simulink model "sampleModel209"  (R2021b)
settings: Solver=VariableStepAuto  StartTime=0.0  StopTime=10.0  RelTol=1e-3
undefined symbols (not defined in the file or in its folder): DiscIntNeverNeededParam, Newton, Raphson
libraries: simulink x2
settings Model: Creator=user  LastModifiedBy=user

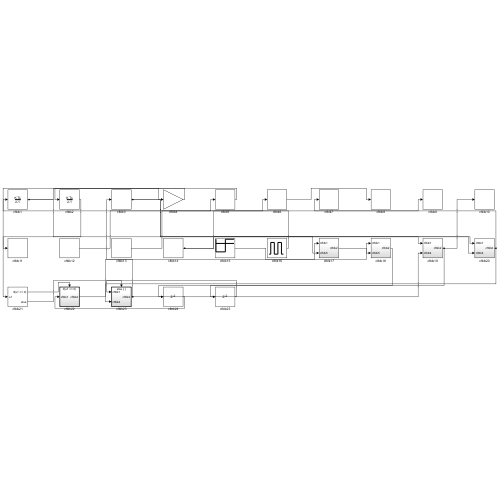
[thumbnail: Simulink's stored preview of the top-level diagram]
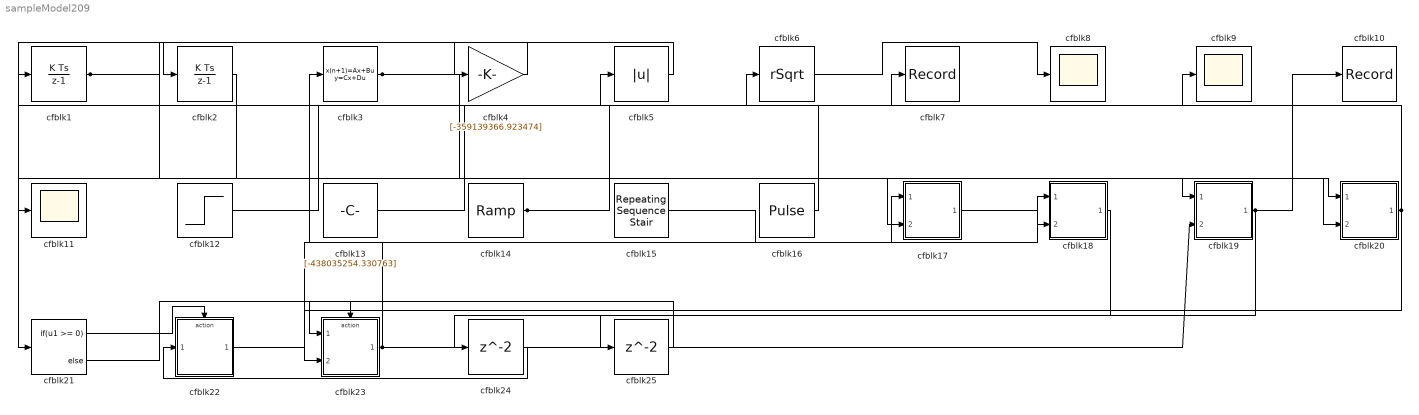
== system sampleModel209 ==
  cfblk1 : DiscreteIntegrator  ICPrevOutput=DiscIntNeverNeededParam  ICPrevScaledInput=DiscIntNeverNeededParam
  cfblk10 : Record  FileSettingsInternal="{\"entries\":[{\"content\":{\"excelSettings\":{\"content\":{},\"type\":\"Streamout.ExcelSettings\"}},\"type\":\"Streamout.FileSettingStorage\",\"uuid\":\"ddcee48c-97f9-4c5e-be8b-3015be74b49a\"}],\"packageUris\":[\"http://schema.mathworks.com/mf0/streamout_blocks/R2020a\"],\"version\":\"1.0\"}"  SignalsInternal="{\"entries\":[{\"content\":{\"signals\":[{\"content\":{\"blockPath\":[\"sampleModel209/cfblk10\"],\"channel\":[],\"dimensions\":[1],\"domain\":\"sampleModel209/cfblk10\",\"lineColor\":\"#ff13a6\",\"plots\":[1],\"port\":1,\"sid\":[\"\"],\"signalID\":8107,\"signalName\":\"cfblk19\"},\"type\":\"RecordBlkView.Signal\",\"uuid\":\"8c198879-0a60-44c0-909a-365ac949948a\"}]},\"type\":\"RecordBlkView.InputSignals\",\"uuid\":\"fa839402-d960-43c3-8ba2-43e0def371db\"}],\"packageUris\":[\"http://schema.mathworks.com/mf0/streamout_blocks/R2020a\"],\"version\":\"1.0\"}"  VisualizationBindings="{\"sparklinesplugin\":{\"info\":[{\"bindingParametersList\":[],\"subplotID\":1}]}}"
  cfblk11 : Scope
  cfblk12 : Step  Time=[34.000000]  Before=[760172402.159032]  After=[340434112.480645]  SampleTime=0
  cfblk13 : Constant  Value=[-438035254.330763]  SampleTime=1
  cfblk14 : simulink/Sources/Ramp  slope=[-6896.997594]  start=[40.335402]  InitialOutput=[-525774.390011]
  cfblk15 : simulink/Sources/Repeating Sequence Stair  OutValues=[-725082246.966305, 369090109.058846]  tsamp=-1  OutMin=[]  OutMax=[]  OutDataTypeStr=double  OutputDataTypeScalingMode=double  OutDataType=fixdt(0,8)  ConRadixGroup=Best Precision: Vector-wise  OutScaling=2^-12
  cfblk16 : DiscretePulseGenerator  PulseType=Time based  Amplitude=[-634459227.469684]  Period=[3400026.159223]  PulseWidth=5  PhaseDelay=[1.000000]
  cfblk17 : Subsystem
  cfblk18 : Subsystem
  cfblk19 : Subsystem
  cfblk2 : DiscreteIntegrator  ICPrevOutput=DiscIntNeverNeededParam  ICPrevScaledInput=DiscIntNeverNeededParam
  cfblk20 : Subsystem
  cfblk21 : If  IfExpression=u1 >= 0  SampleTime=1
  cfblk22 : Subsystem  TreatAsAtomicUnit=on
  cfblk23 : Subsystem  TreatAsAtomicUnit=on
  cfblk24 : Delay  SampleTime=1
  cfblk25 : Delay  SampleTime=1
  cfblk3 : DiscreteStateSpace
  cfblk4 : Gain  Gain=[-359139366.923474]
  cfblk5 : Abs
  cfblk6 : Sqrt  Operator=rSqrt  AlgorithmType=Newton-Raphson  SaturateOnIntegerOverflow=on
  cfblk7 : Record  FileSettingsInternal="{\"entries\":[{\"content\":{\"excelSettings\":{\"content\":{},\"type\":\"Streamout.ExcelSettings\"}},\"type\":\"Streamout.FileSettingStorage\",\"uuid\":\"78a27359-255d-4437-ae35-127f47ed64b3\"}],\"packageUris\":[\"http://schema.mathworks.com/mf0/streamout_blocks/R2020a\"],\"version\":\"1.0\"}"  SignalsInternal="{\"entries\":[{\"content\":{\"signals\":[{\"content\":{\"blockPath\":[\"sampleModel209/cfblk7\"],\"channel\":[],\"dimensions\":[1],\"domain\":\"sampleModel209/cfblk7\",\"lineColor\":\"#fe330a\",\"plots\":[1],\"port\":1,\"sid\":[\"\"],\"signalID\":8111,\"signalName\":\"cfblk20\"},\"type\":\"RecordBlkView.Signal\",\"uuid\":\"cc093a5e-f450-4358-995f-cba163aa30d8\"}]},\"type\":\"RecordBlkView.InputSignals\",\"uuid\":\"e5813685-5132-4ee3-bc5a-e7e5b18a0bcd\"}],\"packageUris\":[\"http://schema.mathworks.com/mf0/streamout_blocks/R2020a\"],\"version\":\"1.0\"}"  VisualizationBindings="{\"sparklinesplugin\":{\"info\":[{\"bindingParametersList\":[],\"subplotID\":1}]}}"
  cfblk8 : Scope
  cfblk9 : Scope
  wires:
  cfblk3/1 -> cfblk19/1(cfblk1), cfblk17/2(cfblk5)
  cfblk13/1 -> cfblk5/1
  cfblk5/1 -> cfblk21/1
  cfblk4/1 -> cfblk2/1
  cfblk15/1 -> cfblk18/1(cfblk1)
  cfblk17/1(cfblk2) -> cfblk18/2(cfblk5)
  cfblk20/1(cfblk2) -> cfblk7/1, cfblk23/2(cfblk4)
  cfblk16/1 -> cfblk1/1
  cfblk2/1 -> cfblk11/1
  cfblk14/1 -> cfblk20/1(cfblk1), cfblk6/1
  cfblk6/1 -> cfblk8/1
  cfblk1/1 -> cfblk20/2(cfblk4), cfblk4/1
  cfblk23/1(cfblk2) -> cfblk19/2(cfblk4), cfblk3/1
  cfblk12/1 -> cfblk9/1
  cfblk22/1(cfblk2) -> cfblk17/1(cfblk1)
  cfblk19/1(cfblk2) -> cfblk10/1, cfblk24/1
  cfblk21/1 -> cfblk22/Action
  cfblk21/2 -> cfblk23/Action
  cfblk24/1 -> cfblk22/1(cfblk1)
  cfblk18/1(cfblk2) -> cfblk25/1
  cfblk25/1 -> cfblk23/1(cfblk1)

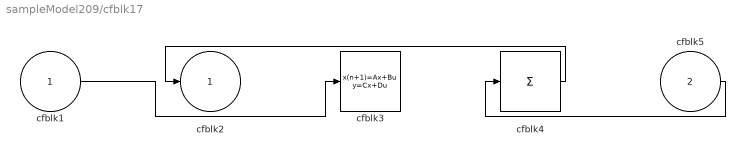
== system sampleModel209/cfblk17 ==
  cfblk1 : Inport
  cfblk5 : Inport  Port=2
  cfblk3 : DiscreteStateSpace
  cfblk4 : Sum  Inputs=+
  cfblk2 : Outport
  wires:
  cfblk4/1 -> cfblk2/1
  cfblk1/1 -> cfblk3/1
  cfblk5/1 -> cfblk4/1

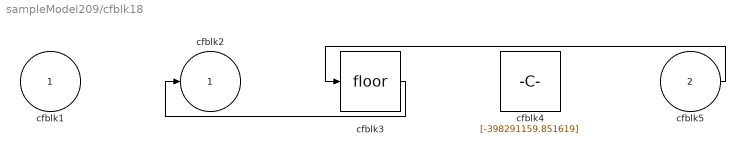
== system sampleModel209/cfblk18 ==
  cfblk1 : Inport
  cfblk5 : Inport  Port=2
  cfblk3 : Rounding
  cfblk4 : Constant  Value=[-398291159.851619]  SampleTime=1
  cfblk2 : Outport
  wires:
  cfblk5/1 -> cfblk3/1
  cfblk3/1 -> cfblk2/1

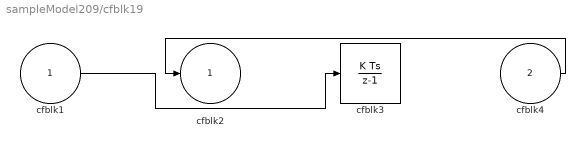
== system sampleModel209/cfblk19 ==
  cfblk1 : Inport
  cfblk4 : Inport  Port=2
  cfblk3 : DiscreteIntegrator  ICPrevOutput=DiscIntNeverNeededParam  ICPrevScaledInput=DiscIntNeverNeededParam
  cfblk2 : Outport
  wires:
  cfblk4/1 -> cfblk2/1
  cfblk1/1 -> cfblk3/1

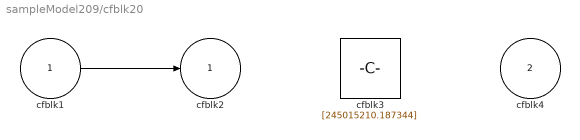
== system sampleModel209/cfblk20 ==
  cfblk1 : Inport
  cfblk4 : Inport  Port=2
  cfblk3 : Constant  Value=[245015210.187344]  SampleTime=1
  cfblk2 : Outport
  wires:
  cfblk1/1 -> cfblk2/1

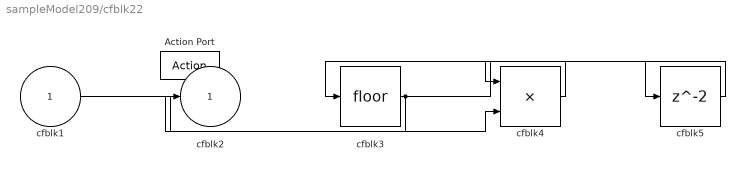
== system sampleModel209/cfblk22 ==
  cfblk1 : Inport
  Action Port : ActionPort  ActionPortLabel=if(u1 >= 0)
  cfblk3 : Rounding
  cfblk4 : Product  Inputs=**
  cfblk5 : Delay
  cfblk2 : Outport
  wires:
  cfblk3/1 -> cfblk2/1, cfblk5/1
  cfblk1/1 -> cfblk4/2
  cfblk4/1 -> cfblk3/1
  cfblk5/1 -> cfblk4/1

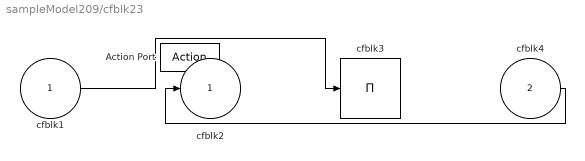
== system sampleModel209/cfblk23 ==
  cfblk1 : Inport
  cfblk4 : Inport  Port=2
  Action Port : ActionPort  ActionPortLabel=else
  cfblk3 : Product  Inputs=*
  cfblk2 : Outport
  wires:
  cfblk4/1 -> cfblk2/1
  cfblk1/1 -> cfblk3/1
